simulink model "StraddleCarrier"  (R2022b)
settings: Solver=FixedStepAuto  StartTime=0  StopTime=1000  FixedStep=Ts  RelTol=1e-3
undefined symbols (not defined in the file): AEB, driving, m, n, q, theta, Ts
libraries: simulink x6, roadrunnerscenario x4, simulink_extras x4, drivingscenarioandsensors x3, uavsim3dlib x3, sim3dprobsensorlib x2, trackingutilitieslib x1, drivinglib x1, sim3dlib x1, sim3dcameralib x1, sim3dphyssensorlib x1, sim3dgroundtruthsensorlib x1
(part 3 of 3)

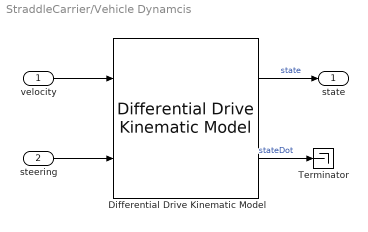
== system StraddleCarrier/Vehicle Dynamcis ==
  velocity : Inport
  steering : Inport  Port=2
  Differential Drive Kinematic Model : robotmobilelib/Differential Drive Kinematic Model  VehicleInputs=Vehicle Speed & Heading Angular Velocity  WheelRadius=3  WheelSpeedRange=[-inf inf]  TrackWidth=3  InitialState=[q(1,1) q(2,1) theta(1)]  SimulateUsing=Interpreted execution
  Terminator : Terminator
  state : Outport
  wires:
  Differential Drive Kinematic Model/2 -> Terminator/1  "stateDot"
  steering/1 -> Differential Drive Kinematic Model/2
  velocity/1 -> Differential Drive Kinematic Model/1
  Differential Drive Kinematic Model/1 -> state/1  "state"

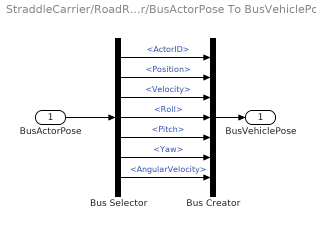
== system StraddleCarrier/RoadRunner Reader/BusActorPose To BusVehiclePose ==
  BusActorPose : Inport
  Bus Creator : BusCreator  Inputs=7  OutDataTypeStr=Bus: BusVehiclePose  NonVirtualBus=on
      settings: InheritFromInputs=off
  Bus Selector : BusSelector  OutputSignals=ActorID,Position,Velocity,Roll,Pitch,Yaw,AngularVelocity
  BusVehiclePose : Outport
  wires:
  BusActorPose/1 -> Bus Selector/1
  Bus Selector/1 -> Bus Creator/1  "<ActorID>"
  Bus Selector/2 -> Bus Creator/2  "<Position>"
  Bus Selector/4 -> Bus Creator/4  "<Roll>"
  Bus Selector/5 -> Bus Creator/5  "<Pitch>"
  Bus Selector/6 -> Bus Creator/6  "<Yaw>"
  Bus Selector/7 -> Bus Creator/7  "<AngularVelocity>"
  Bus Selector/3 -> Bus Creator/3  "<Velocity>"
  Bus Creator/1 -> BusVehiclePose/1

== system StraddleCarrier/RoadRunner Writer/BusVehiclePose To BusActorPose ==
  BusVehiclePose : Inport
  Bus Creator : BusCreator  Inputs=7  OutDataTypeStr=Bus: BusActorPose  NonVirtualBus=on
      settings: InheritFromInputs=off
  Bus Selector : BusSelector  OutputSignals=ActorID,Position,Velocity,Roll,Pitch,Yaw,AngularVelocity
  BusActorPose : Outport
  wires:
  BusVehiclePose/1 -> Bus Selector/1
  Bus Selector/1 -> Bus Creator/1  "<ActorID>"
  Bus Selector/2 -> Bus Creator/2  "<Position>"
  Bus Selector/4 -> Bus Creator/4  "<Roll>"
  Bus Selector/5 -> Bus Creator/5  "<Pitch>"
  Bus Selector/6 -> Bus Creator/6  "<Yaw>"
  Bus Selector/7 -> Bus Creator/7  "<AngularVelocity>"
  Bus Selector/3 -> Bus Creator/3  "<Velocity>"
  Bus Creator/1 -> BusActorPose/1

== matlab function StraddleCarrier/Unreal Engine Sensors/Visualize Point cloud ==
  data: xyzPoints input
function VisualizePointCloud(xyzPoints)
%VisualizePointCloud Display point cloud

coder.extrinsic('isOpen', 'pcplayer')

persistent player;

if isempty(player)
    % Configure axes limits
    xlimits = [-90 90];
    ylimits = [-90 90];
    zlimits = [ -5 40];
    
    % Create a streaming Lidar viewer
    player = pcplayer(xlimits, ylimits, zlimits);
end

if ~isempty(player) && isOpen(player)
    view(player, xyzPoints);
end

== matlab function StraddleCarrier/Autonomous Emergency Brake/AEB Logics ==
  data: Tracks input Bus: BusMultiObjectTracker1; AEB output boolean size=[1 1]; threshold input; numTracks output; distance output
function [AEB, numTracks, distance] = findLeadCar(Tracks, threshold)

persistent tmpStop
if isempty(tmpStop)
    tmpStop = false;
end

x = 0;
y = 0;
dis = 99999;
numTracks = Tracks.NumTracks;
distance = 99999;

for i = 1 : numTracks
    x = Tracks.Tracks(i).State(1);
    y = Tracks.Tracks(i).State(3);
    dis = sqrt(x*x + y*y);
    
    if dis < distance
        distance = dis;
    end

    if dis < threshold
        tmpStop = true;
        distance = dis;
        break
    end
end

AEB = tmpStop;

end

== matlab function StraddleCarrier/RoadRunner Writer/Pack Ego Actor2 ==
  data: pos input; Pose output Bus: BusVehiclePose size=1; vel input; yaw input; yawRate input; egoActorID parameter
function Pose = packEgo(pos,vel,yaw,yawRate, egoActorID)
% Pack ego information into a single ego actor bus
%
% Important note:
% Output is a bus of type BusVehiclePose. This bus must match the bus 
% elements expected by Scenario Reader. You can view the 
% bus association using 'Edit Data' in the menu above.

Pose = struct(...
    'ActorID', egoActorID,...
    'Position', [pos(1) pos(2) 0], ...
    'Velocity', [vel(1) vel(2) 0], ...
    'Roll', 0, ...
    'Pitch', 0, ...
    'Yaw', yaw, ...
    'AngularVelocity', [0 0 yawRate]);
